simulink model "productionLine_2Machines"  (R2024b)
settings: Solver=VariableStepAuto  StartTime=0.0  StopTime=100  RelTol=1e-3
model workspace (MAT data in the model file):
  bufferCapacity1 = 50
  bufferProcessedProducts = 50
undefined symbols (not defined in the file): m, n
libraries: rllib x1
settings Model: SimulationMode=accelerator  Creator=giopa  LastModifiedBy=giopa

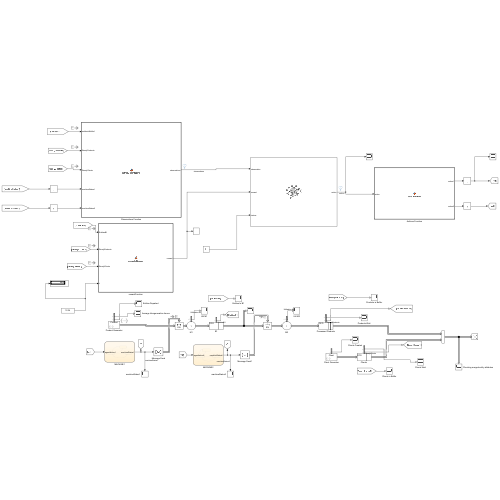
[thumbnail: Simulink's stored preview of the top-level diagram]
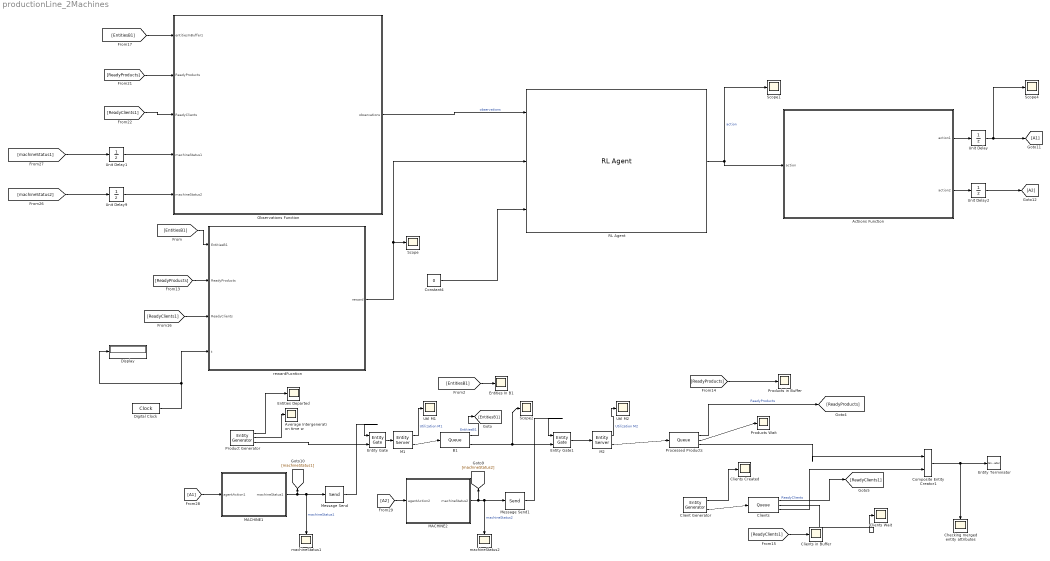
== system productionLine_2Machines ==
  Actiions Function : MATLAB Function  TreatAsAtomicUnit=on
  Average Intergeneration time w : Scope
  B1 : Queue  InputPortMessageModes=m  OutputPortMessageModes=n,m  Capacity=bufferCapacity1  NumberEntitiesInBlock=on
      settings: OutputPortMap=o1,o5
  Checking merged entity attributes : Scope
  Client Generator : EntityGenerator  OutputPortMessageModes=n,m  TimeSource=MATLAB action  IntergenerationTimeAction=|  GenerateEntityAtSimulationStart=off  GenerateAction=|  AttributeName=clientNumber  NumberEntitiesDeparted=on  EntityType=Structured  EntityTypeName=Client
      IntergenerationTimeAction=|
      | muI = 4.5;   % Mean intergeneration time 
      | dt = -muI * log(1 - rand());  % Exponential distribution
      GenerateAction=|
      | persistent clientNumber;
      | if isempty(clientNumber)
      |     clientNumber = 0; % Initialize the first client number
      | else
      |     clientNumber = clientNumber + 1; % Increment client number for each new entity
      | end
      | entity.clientNumber = clientNumber; % Assign the number to the entity's attribute
      settings: OutputPortMap=o0,o3
  "Clients " : Queue  InputPortMessageModes=m  OutputPortMessageModes=n,n,m  Capacity=50  NumberEntitiesInBlock=on  AverageWait=on
      settings: OutputPortMap=o1,o2,o5
  Clients Created : Scope
  Clients Wait : Scope
  Clients in Buffer : Scope
  Composite Entity Creator1 : CompositeEntityCreator  InputPortMessageModes=m,m  OutputPortMessageModes=m  EntityTypeName=Order  InputEntityName=Product|Client
      settings: InputPortMap=u0,u1
  Constant4 : Constant  Value=0
  Digital Clock : DigitalClock  SampleTime=0.1
  Display : Display
  Entities Departed : Scope
  Entities In B1 : Scope
  Entity Gate : EntityGate  InputPortMessageModes=m,m  OutputPortMessageModes=m  MatchingAttributeName=gateCheck  InitialValueOfMatchingAttribute=1  OpenGateAtSimulationStart=on
  Entity Gate1 : EntityGate  InputPortMessageModes=m,m  OutputPortMessageModes=m  MatchingAttributeName=machineStatus  InitialValueOfMatchingAttribute=1
  Entity Terminator : EntityTerminator  InputPortMessageModes=m
  M1 : EntityServer  InputPortMessageModes=m  OutputPortMessageModes=n,m  Capacity=1  ServiceTimeSource=Attribute  ServiceTimeValue=1  ServiceTimeAttributeName=processingTime  Utilization=on
      settings: OutputPortMap=o5,o9
  M2 : EntityServer  InputPortMessageModes=m  OutputPortMessageModes=n,m  Capacity=1  ServiceTimeSource=Attribute  ServiceTimeValue=1  ServiceTimeAttributeName=processingTime  Utilization=on
      settings: OutputPortMap=o5,o9
  MACHINE1 : Stateflow chart  TreatAsAtomicUnit=on
  MACHINE2 : Stateflow chart  TreatAsAtomicUnit=on
  Message Send : Send  OutputPortMessageModes=m
  Message Send1 : Send  OutputPortMessageModes=m
  Observations Function : MATLAB Function  TreatAsAtomicUnit=on
  Processed Products : Queue  InputPortMessageModes=m  OutputPortMessageModes=n,n,m  Capacity=bufferProcessedProducts  NumberEntitiesInBlock=on  AverageWait=on
      settings: OutputPortMap=o1,o2,o5
  Product Generator : EntityGenerator  OutputPortMessageModes=n,n,m  Period=2.7  IntergenerationTimeAction=|  GenerateAction=|  ExitAction=|  AttributeName=processingTime|productNumber|entryTime  AttributeInitialValue=2|1|1  NumberEntitiesDeparted=on  AverageIntergenerationTime=on  EntityType=Structured  EntityTypeName=Product
      IntergenerationTimeAction=|
      | muI = 2;   % Mean intergeneration time 
      | dt = -muI * log(1 - rand());  % Exponential distribution
      GenerateAction=|
      | persistent rngInit;
      | if isempty(rngInit)
      |     seed = 12345;
      |     rng(seed);
      |     rngInit = true;
      | end
      | % Pattern: Exponential distribution
      | 
      | mu = 2;
      | entity.processingTime = -mu * log(1 - rand());
      | 
      | %assign productNumber aatribute to every entity
      | persistent productNumber
      | if isempty(productNumber)
      |     productNumber = 0;  
      | end
      | 
      | % Assign productNumber attribute
      | entity.productNumber = productNumber + 1; % Increment and assign the product number
      | productNumber = productNumber + 1;        % Update the product number for the next product
      ExitAction=|
      | persistent productNumber;
      | if isempty(productNumber)
      |     productNumber = 1; % Initialize the first client number
      | else
      |     productNumber = productNumber + 1; % Increment client number for each new entity
      | end
      | entity.productNumber = productNumber; % Assign the number to the entity's attribute
      settings: OutputPortMap=o0,o2,o3
  Products Wait : Scope
  Products in Buffer : Scope
  RL Agent : rllib/RL Agent  Agent=agent  ExternalActionAsInput=off  ProvideLastAction=off  ProvideCumRwd=off  TreatAsDirectFeedthrough=on  UseStrictObservationDataTypes=off
  Scope{,1..2,4} (4 alike) : Scope
  Unit Delay : UnitDelay  SampleTime=-1  HasFrameUpgradeWarning=on
  Unit Delay1 : UnitDelay  InitialCondition=1  SampleTime=-1  HasFrameUpgradeWarning=on
  Unit Delay2 : UnitDelay  SampleTime=-1  HasFrameUpgradeWarning=on
  Unit Delay9 : UnitDelay  InitialCondition=1  SampleTime=-1  HasFrameUpgradeWarning=on
  Util M1 : Scope
  Util M2 : Scope
  machineStatus1 : Scope
  machineStatus2 : Scope
  rewardFucntion : MATLAB Function  TreatAsAtomicUnit=on
  wires:
  RL Agent/1 -> Scope1/1, Actiions Function/1(action)  "action"
  Message Send1/1 -> Entity Gate1/1
  rewardFucntion/1(reward) -> Scope/1, RL Agent/2
  "Clients "/3 -> Composite Entity Creator1/2
  Client Generator/1 -> Clients Created/1
  [machineStatus1] -> Unit Delay1/1
  [EntitiesB1] -> rewardFucntion/1(EntitiesB1)
  "Clients "/2 -> Clients Wait/1
  Processed Products/2 -> Products Wait/1
  Product Generator/2 -> Average Intergeneration time w/1
  [ReadyClients1] -> Clients in Buffer/1
  [A1] -> MACHINE1/1(agentAction1)
  [ReadyClients1] -> rewardFucntion/3(ReadyClients)
  Product Generator/3 -> Entity Gate/2
  [ReadyProducts] -> Observations Function/2(ReadyProducts)
  Unit Delay2/1 -> [A2]
  M1/2 -> B1/1
  Actiions Function/1(action1) -> Unit Delay/1
  B1/2 -> Scope2/1, Entity Gate1/2
  [ReadyProducts] -> Products in Buffer/1
  [A2] -> MACHINE2/1(agentAction2)
  Composite Entity Creator1/1 -> Entity Terminator/1, Checking merged entity attributes/1
  [machineStatus2] -> Unit Delay9/1
  Processed Products/1 -> [ReadyProducts]  "ReadyProducts"
  Digital Clock/1 -> Display/1, rewardFucntion/4(t)
  Entity Gate/1 -> M1/1
  [EntitiesB1] -> Observations Function/1(entitiesInBuffer1)
  Actiions Function/2(action2) -> Unit Delay2/1
  "Clients "/1 -> [ReadyClients1]  "ReadyClients"
  M2/2 -> Processed Products/1
  M1/1 -> Util M1/1  "Utilization M1"
  Product Generator/1 -> Entities Departed/1
  B1/1 -> [EntitiesB1]  "EntitiesB1"
  Processed Products/3 -> Composite Entity Creator1/1
  M2/1 -> Util M2/1  "Utilization M2"
  Client Generator/2 -> "Clients "/1
  Unit Delay9/1 -> Observations Function/5(machineStatus2)
  [ReadyClients1] -> Observations Function/3(ReadyClients)
  [ReadyProducts] -> rewardFucntion/2(ReadyProducts)
  MACHINE2/1(machineStatus2) -> [machineStatus2], machineStatus2/1, Message Send1/1  "machineStatus2"
  Unit Delay/1 -> Scope4/1, [A1]
  Observations Function/1(observations) -> RL Agent/1  "observations"
  [EntitiesB1] -> Entities In B1/1
  Constant4/1 -> RL Agent/3
  MACHINE1/1(machineStatus1) -> machineStatus1/1, Message Send/1, [machineStatus1]  "machineStatus1"
  Entity Gate1/1 -> M2/1
  Unit Delay1/1 -> Observations Function/4(machineStatus1)
  Message Send/1 -> Entity Gate/1

== matlab function productionLine_2Machines/Actiions Function ==
  data: action input; action1 output; action2 output
function [action1, action2] = decodeAction(action)
    % Ensure action is treated as a numeric array
    % Directly use action as a numeric vector

    % Assign each binary digit to the respective machine's action
    action1 = action(1);  % Action for Machine 1
    action2 = action(2);  % Action for Machine 2
end

== stateflow chart productionLine_2Machines/MACHINE2 ==
  state Failed
    entry:
    machineStatus2 = 0;
    repairTime2 = -meanRepairTime2 * log(1 - rand());
  state Idle
    entry:
    machineStatus2 = -1;
  state Working
    entry:
    machineStatus2 = 1;
    timeToFailure2 = -meanFailureTime2 * log(1 - rand());
  Working -> Failed [order 1] : [after(timeToFailure2, sec)]
  Failed -> Working : [after(repairTime2, sec)]
  (default) -> Working
  Idle -> Working : [agentAction2 == 1]
  Working -> Idle [order 2] : [agentAction2 == 0]
  data: meanRepairTime2 constant double =5; meanFailureTime2 constant double =50; machineStatus2 output; repairTime2 local; timeToFailure2 local; agentAction2 input

== stateflow chart productionLine_2Machines/MACHINE1 ==
  state Failed
    entry:
    machineStatus1 = 0;
    repairTime1 = -meanRepairTime1 * log(1 - rand());
  state Idle
    entry:
    machineStatus1 = -1;
  state Working
    entry:
    machineStatus1 = 1;
    timeToFailure1 = -meanFailureTime1 * log(1 - rand());
  Working -> Failed [order 1] : [after(timeToFailure1, sec)]
  Failed -> Working : [after(repairTime1, sec)]
  (default) -> Working
  Idle -> Working : [agentAction1 == 1]
  Working -> Idle [order 2] : [agentAction1 == 0]
  data: meanRepairTime1 constant double =5; meanFailureTime1 constant double =50; machineStatus1 output; repairTime1 local; timeToFailure1 local; agentAction1 input

== matlab function productionLine_2Machines/Observations Function ==
  data: entitiesInBuffer1 input; observations output; ReadyProducts input; ReadyClients input; machineStatus1 input; machineStatus2 input
function observations = gatherObservations(entitiesInBuffer1, ReadyProducts, ReadyClients, ...
                                           machineStatus1, machineStatus2)
    % Define maximum buffer capacity
    maxBufferCapacity = 50;

    % Normalize buffer level
    bufferLevels = entitiesInBuffer1 / maxBufferCapacity;

    % Normalize ready products and clients
    readyStates = [ReadyProducts; ReadyClients] / maxBufferCapacity;

    % Normalize machine states to [0, 1]
    machineStates = [machineStatus1; machineStatus2];

    % Combine normalized observations into a single vector
    observations = [bufferLevels; readyStates; machineStates];
end

== matlab function productionLine_2Machines/rewardFucntion ==
  data: EntitiesB1 input; ReadyProducts input; ReadyClients input; reward output; t input
function reward = calculateReward(EntitiesB1, ReadyProducts, ReadyClients, t)
    % Time tracking
    persistent lastTime
    if isempty(lastTime)
        lastTime = t;
        reward = 0;
        return;
    end

    % Calculate time step
    dt = t - lastTime;
    lastTime = t;

    % Cost weights (adjusted for 2-machine setup)
    bufferCost = 0.5;      % Cost for entities in Buffer B1
    productsCost = 1;      % Cost for products waiting after processing
    clientsCost = 1.3;     % Cost for clients waiting before merging

    % Calculate total cost
    totalCost = (EntitiesB1 * bufferCost + ReadyProducts * productsCost + ReadyClients * clientsCost) * dt;

    % Reward is the negative total cost (to encourage minimization)
    reward = -totalCost;
end
